simulink model "DemoCommentsModel"  (R2024a)
settings: Solver=VariableStepAuto  StartTime=0.0  StopTime=10.0  RelTol=1e-3
undefined symbols (not defined in the file or in its folder): m, magnitude
settings Model: Creator=chris  LastModifiedBy=chris

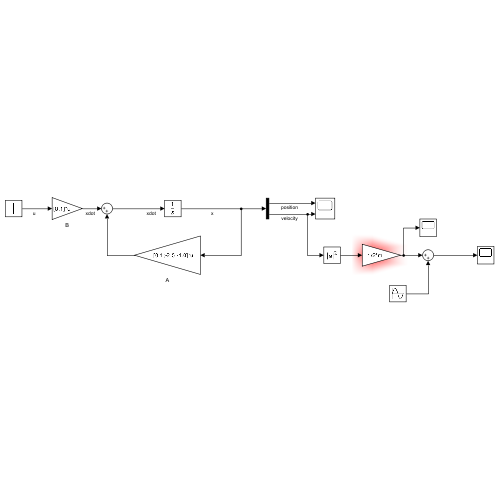
[thumbnail: Simulink's stored preview of the top-level diagram]
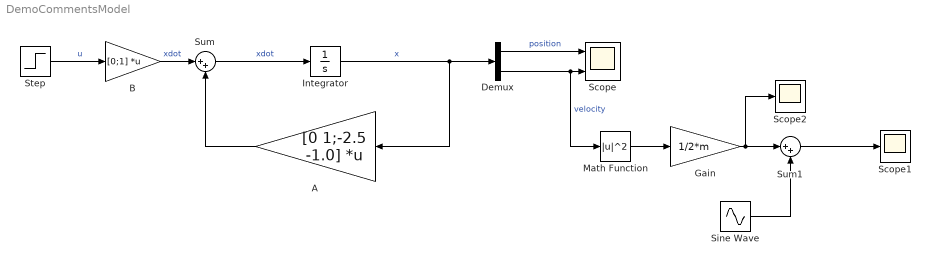
== system DemoCommentsModel ==
  A : Gain  Gain=[0 1;-2.5 -1.0]  Multiplication=Matrix(K*u)
  B : Gain  Gain=[0;1]  Multiplication=Matrix(K*u)
  Demux : Demux  Outputs=2
  Gain : Gain  Gain=1/2*m
  Integrator : Integrator
  Math Function : Math  Operator=magnitude^2
  Scope : Scope  NumInputPorts=2
  Scope1 : Scope
  Scope2 : Scope
  Sine Wave : Sin  Amplitude=.01  Frequency=2  SampleTime=0
  Step : Step  SampleTime=0
  Sum : Sum  Inputs=|++
  Sum1 : Sum  Inputs=|++
  wires:
  Sum/1 -> Integrator/1  "xdot"
  Integrator/1 -> Demux/1, A/1  "x"
  A/1 -> Sum/2
  B/1 -> Sum/1  "xdot"
  Step/1 -> B/1  "u"
  Demux/2 -> Math Function/1, Scope/2  "velocity"
  Demux/1 -> Scope/1  "position"
  Math Function/1 -> Gain/1
  Gain/1 -> Scope2/1, Sum1/1
  Sine Wave/1 -> Sum1/2
  Sum1/1 -> Scope1/1
